simulink model "Deliverable2_SimulinkModel_Group37_Demo"  (R2023b)
settings: Solver=FixedStepAuto  StartTime=0.0  StopTime=10.0  RelTol=1e-3  EnableMultiTasking=on
undefined symbols (not defined in the file): A0, A1, D0, D1, D10, D11, D12, D13, D2, D3, D4, D5, D6, D7, D8, D9, PTA0, PTA1, PTA2, PTB2, PTB23, PTB3, PTB9, PTC16, PTC17, PTC2, PTC3, PTC4, PTD0, PTD1, PTD2, PTD3, send_params
libraries: frdmk64flib x20, etargetslib x2, simulink x2
settings Model: ExtModeTrigDuration=5  Creator=cakes  LastModifiedBy=cakes
settings OptimizationCC: EnhancedBackFolding=on  PassReuseOutputArgsAs=Individual arguments  ZeroExternalMemoryAtStartup=off  ZeroInternalMemoryAtStartup=off  MaxStackSize=64  OptimizeBlockOrder=speed  DifferentSizesBufferReuse=on  OptimizationCustomize=off  EfficientTunableParamExpr=on
settings DebuggingCC: ParameterTunabilityLossMsg=error
settings HardwareCC: ProdBitPerPointer=32  ProdBitPerSizeT=32  ProdBitPerPtrDiffT=32  ProdLargestAtomicInteger=Long  ProdLargestAtomicFloat=Double  ProdWordSize=32  ProdHWDeviceType=ARM Compatible->ARM Cortex
settings SFSimCC: MATLABDynamicMemAlloc=off
settings RTWCC: Description=Embedded Coder  SystemTargetFile=ert.tlc  HardwareBoard=NXP FRDM-K64F  TLCOptions="-aInlineSetEventsForThisBaseRateFcn=TLC_FALSE -aSuppressMultiTaskScheduler=TLC_FALSE  -aRateBasedStepFcn=0"  TemplateMakefile=ert_default_tmf  Toolchain=GNU Tools for ARM Embedded Processors
settings CodeAppCC: ForceParamTrailComments=on  IgnoreCustomStorageClasses=off  OperatorAnnotations=on  SimulinkDataObjDesc=on  SFDataObjDesc=on  InsertBlockDesc=on
settings ERTTargetCC: ExtModeTransport=4  ExtModeMexFile=sendToCommService

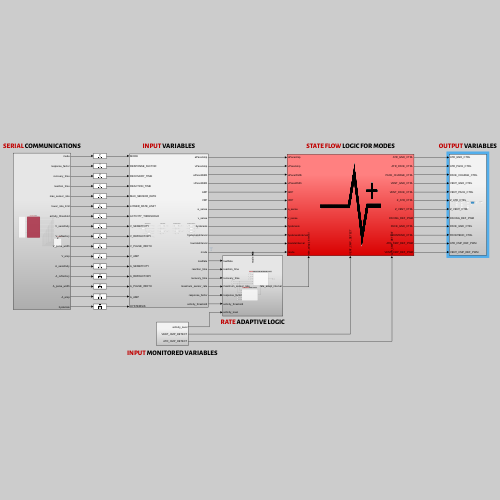
[thumbnail: Simulink's stored preview of the top-level diagram]
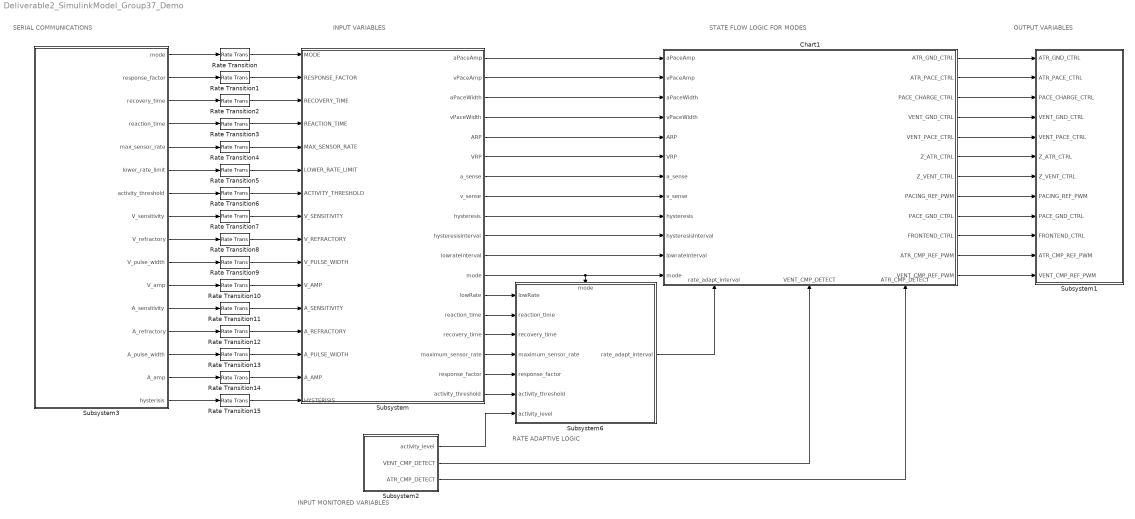
== system Deliverable2_SimulinkModel_Group37_Demo ==
  note: STATE FLOW LOGIC FOR MODES
  note: INPUT VARIABLES
  note: OUTPUT VARIABLES
  note: INPUT MONITORED VARIABLES
  note: SERIAL COMMUNICATIONS
  note: RATE ADAPTIVE LOGIC
  Chart1 : Stateflow chart  TreatAsAtomicUnit=on
      settings: PortSchema="{\"entries\":[{\"content\":{\"sides\":[{\"content\":{\"connectorIds\":[\"In3\",\"In4\",\"In5\",\"In6\",\"In7\",\"In8\",\"In10\",\"In11\",\"In14\",\"In13\",\"In9\",\"In12\"]},\"type\":\"ConnectorPlacement.EquallySpacedRectSide\",\"uuid\":\"0645b224-ea0f-4252-ab3f-59541b69d578\"},{\"content\":{\"connectorIds\":[\"Out1\",\"Out2\",\"Out3\",\"Out4\",\"Out5\",\"Out6\",\"Out7\",\"Out8\",\"Out9\",\"Out10\",\"Out12\",\"Out11\"],\"side\":\"RIGHT\"},\"type\":\"ConnectorPlacement.EquallySpacedRectSide\",\"uuid\":\"774839c9-1eb4-4ab6-be6e-099c2bb8a485\"},{\"content\":{\"side\":\"TOP\"},\"type\":\"ConnectorPlacement.EquallySpacedRectSide\",\"uuid\":\"6cb60565-1780-4b9d-884d-75d2ba8c5024\"},{\"content\":{\"connectorIds\":[\"In15\",\"In1\",\"In2\"],\"side\":\"BOTTOM\"},\"type\":\"ConnectorPlacement.EquallySpacedRectSide\",\"uuid\":\"cb44bc08-16a9-4dba-a42a-7ec56f3e5fd4\"}]},\"type\":\"ConnectorPlacement.EquallySpacedConnector\",\"uuid\":\"755e29d5-bc4e-404e-b866-950d5e4fdc89\"}],\"packageUris\":[\"http://schema.mathworks.com/mf0/Connector/R2020b\"],\"version\":\"1.0\"}"
  Rate Transition{,1..15} (16 alike) : RateTransition  OutPortSampleTime=0.001
  Subsystem : Subsystem
  Subsystem1 : Subsystem
  Subsystem2 : Subsystem
  Subsystem3 : Subsystem
  Subsystem6 : Subsystem
      settings: PortSchema="{\"entries\":[{\"content\":{\"sides\":[{\"content\":{\"connectorIds\":[\"In1\",\"In2\",\"In3\",\"In4\",\"In5\",\"In6\",\"In7\"]},\"type\":\"ConnectorPlacement.EquallySpacedRectSide\",\"uuid\":\"e8f7da03-bd10-42b0-9ffd-e59584e5bdf1\"},{\"content\":{\"connectorIds\":[\"Out1\"],\"side\":\"RIGHT\"},\"type\":\"ConnectorPlacement.EquallySpacedRectSide\",\"uuid\":\"86778467-52ef-4ae1-a721-8cc17c3ab00e\"},{\"content\":{\"connectorIds\":[\"In8\"],\"side\":\"TOP\"},\"type\":\"ConnectorPlacement.EquallySpacedRectSide\",\"uuid\":\"0329b3a8-8570-41f7-8001-3ae6aa58e01f\"}]},\"type\":\"ConnectorPlacement.EquallySpacedConnector\",\"uuid\":\"40165bd5-ab6e-4098-a980-e92209030f0d\"}],\"packageUris\":[\"http://schema.mathworks.com/mf0/Connector/R2020b\"],\"version\":\"1.0\"}"
  wires:
  Subsystem/1(aPaceAmp) -> Chart1/3(aPaceAmp)
  Subsystem/2(vPaceAmp) -> Chart1/4(vPaceAmp)
  Subsystem/3(aPaceWidth) -> Chart1/5(aPaceWidth)
  Subsystem/4(vPaceWidth) -> Chart1/6(vPaceWidth)
  Subsystem/5(ARP) -> Chart1/7(ARP)
  Subsystem/6(VRP) -> Chart1/8(VRP)
  Subsystem/11(lowrateInterval) -> Chart1/9(lowrateInterval)
  Subsystem/12(mode) -> Subsystem6/8(mode), Chart1/12(mode)
  Chart1/1(ATR_GND_CTRL) -> Subsystem1/1(ATR_GND_CTRL)
  Chart1/2(ATR_PACE_CTRL) -> Subsystem1/2(ATR_PACE_CTRL)
  Chart1/3(PACE_CHARGE_CTRL) -> Subsystem1/3(PACE_CHARGE_CTRL)
  Chart1/4(VENT_GND_CTRL) -> Subsystem1/4(VENT_GND_CTRL)
  Chart1/5(VENT_PACE_CTRL) -> Subsystem1/5(VENT_PACE_CTRL)
  Chart1/6(Z_ATR_CTRL) -> Subsystem1/6(Z_ATR_CTRL)
  Subsystem2/2(VENT_CMP_DETECT) -> Chart1/1(VENT_CMP_DETECT)
  Chart1/9(PACE_GND_CTRL) -> Subsystem1/9(PACE_GND_CTRL)
  Subsystem/7(a_sense) -> Chart1/10(a_sense)
  Subsystem/8(v_sense) -> Chart1/11(v_sense)
  Chart1/10(FRONTEND_CTRL) -> Subsystem1/10(FRONTEND_CTRL)
  Chart1/11(VENT_CMP_REF_PWM) -> Subsystem1/12(VENT_CMP_REF_PWM)
  Chart1/7(Z_VENT_CTRL) -> Subsystem1/7(Z_VENT_CTRL)
  Chart1/8(PACING_REF_PWM) -> Subsystem1/8(PACING_REF_PWM)
  Chart1/12(ATR_CMP_REF_PWM) -> Subsystem1/11(ATR_CMP_REF_PWM)
  Subsystem2/3(ATR_CMP_DETECT) -> Chart1/2(ATR_CMP_DETECT)
  Subsystem/9(hysteresis) -> Chart1/14(hysteresis)
  Subsystem/10(hysteresisInterval) -> Chart1/13(hysteresisInterval)
  Subsystem/17(response_factor) -> Subsystem6/5(response_factor)
  Subsystem/16(maximum_sensor_rate) -> Subsystem6/4(maximum_sensor_rate)
  Subsystem/13(lowRate) -> Subsystem6/1(lowRate)
  Subsystem/14(reaction_time) -> Subsystem6/2(reaction_time)
  Subsystem/15(recovery_time) -> Subsystem6/3(recovery_time)
  Subsystem/18(activity_threshold) -> Subsystem6/6(activity_threshold)
  Subsystem6/1(rate_adapt_interval) -> Chart1/15(rate_adapt_interval)
  Subsystem2/1(activity_level) -> Subsystem6/7(activity_level)
  Subsystem3/1(mode) -> Rate Transition/1
  Subsystem3/2(response_factor) -> Rate Transition1/1
  Subsystem3/3(recovery_time) -> Rate Transition2/1
  Subsystem3/4(reaction_time) -> Rate Transition3/1
  Subsystem3/5(max_sensor_rate) -> Rate Transition4/1
  Subsystem3/7(activity_threshold) -> Rate Transition6/1
  Subsystem3/8(V_sensitivity) -> Rate Transition7/1
  Subsystem3/9(V_refractory) -> Rate Transition8/1
  Subsystem3/10(V_pulse_width) -> Rate Transition9/1
  Subsystem3/14(A_pulse_width) -> Rate Transition13/1
  Subsystem3/13(A_refractory) -> Rate Transition12/1
  Subsystem3/12(A_sensitivity) -> Rate Transition11/1
  Subsystem3/11(V_amp) -> Rate Transition10/1
  Subsystem3/15(A_amp) -> Rate Transition14/1
  Subsystem3/16(hysterisis) -> Rate Transition15/1
  Subsystem3/6(lower_rate_limit) -> Rate Transition5/1
  Rate Transition/1 -> Subsystem/1(MODE)
  Rate Transition1/1 -> Subsystem/2(RESPONSE_FACTOR)
  Rate Transition3/1 -> Subsystem/4(REACTION_TIME)
  Rate Transition2/1 -> Subsystem/3(RECOVERY_TIME)
  Rate Transition4/1 -> Subsystem/5(MAX_SENSOR_RATE)
  Rate Transition5/1 -> Subsystem/6(LOWER_RATE_LIMIT)
  Rate Transition7/1 -> Subsystem/8(V_SENSITIVITY)
  Rate Transition6/1 -> Subsystem/7(ACTIVITY_THRESHOLD)
  Rate Transition9/1 -> Subsystem/10(V_PULSE_WIDTH)
  Rate Transition8/1 -> Subsystem/9(V_REFRACTORY)
  Rate Transition11/1 -> Subsystem/12(A_SENSITIVITY)
  Rate Transition10/1 -> Subsystem/11(V_AMP)
  Rate Transition13/1 -> Subsystem/14(A_PULSE_WIDTH)
  Rate Transition14/1 -> Subsystem/15(A_AMP)
  Rate Transition12/1 -> Subsystem/13(A_REFRACTORY)
  Rate Transition15/1 -> Subsystem/16(HYSTERISIS)

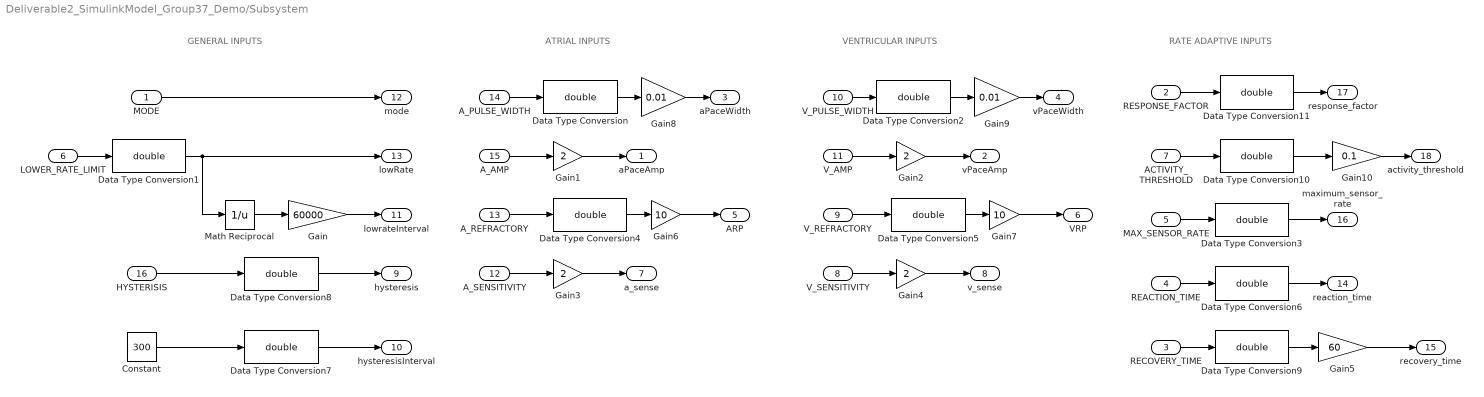
== system Deliverable2_SimulinkModel_Group37_Demo/Subsystem ==
  note: GENERAL INPUTS
  note: ATRIAL INPUTS
  note: VENTRICULAR INPUTS
  note: RATE ADAPTIVE INPUTS
  MODE : Inport
  RESPONSE_FACTOR : Inport  Port=2
  RECOVERY_TIME : Inport  Port=3
  REACTION_TIME : Inport  Port=4
  MAX_SENSOR_RATE : Inport  Port=5
  LOWER_RATE_LIMIT : Inport  Port=6
  ACTIVITY_THRESHOLD : Inport  Port=7
  V_SENSITIVITY : Inport  Port=8
  V_REFRACTORY : Inport  Port=9
  V_PULSE_WIDTH : Inport  Port=10
  V_AMP : Inport  Port=11
  A_SENSITIVITY : Inport  Port=12
  A_REFRACTORY : Inport  Port=13
  A_PULSE_WIDTH : Inport  Port=14
  A_AMP : Inport  Port=15
  HYSTERISIS : Inport  Port=16
  Constant : Constant  Value=300
  Data Type Conversion{,1..11} (12 alike) : DataTypeConversion  OutDataTypeStr=double  SaturateOnIntegerOverflow=off  RndMeth=Floor
  Gain : Gain  Gain=60000
  Gain1 : Gain  Gain=2  OutDataTypeStr=double
  Gain10 : Gain  Gain=0.1  OutDataTypeStr=double
  Gain2 : Gain  Gain=2  OutDataTypeStr=double
  Gain3 : Gain  Gain=2
  Gain4 : Gain  Gain=2
  Gain5 : Gain  Gain=60  OutDataTypeStr=double
  Gain6 : Gain  Gain=10  OutDataTypeStr=double
  Gain7 : Gain  Gain=10  OutDataTypeStr=double
  Gain8 : Gain  Gain=0.01  OutDataTypeStr=double
  Gain9 : Gain  Gain=0.01  OutDataTypeStr=double
  Math Reciprocal : Math  Operator=reciprocal  SignedPower=on
  aPaceAmp : Outport
  vPaceAmp : Outport  Port=2
  aPaceWidth : Outport  Port=3
  vPaceWidth : Outport  Port=4
  ARP : Outport  Port=5
  VRP : Outport  Port=6
  a_sense : Outport  Port=7
  v_sense : Outport  Port=8
  hysteresis : Outport  Port=9
  hysteresisInterval : Outport  Port=10
  lowrateInterval : Outport  Port=11
  mode : Outport  Port=12
  lowRate : Outport  Port=13
  reaction_time : Outport  Port=14
  recovery_time : Outport  Port=15
  maximum_sensor_rate : Outport  Port=16
  response_factor : Outport  Port=17
  activity_threshold : Outport  Port=18
  wires:
  A_PULSE_WIDTH/1 -> Data Type Conversion/1
  V_PULSE_WIDTH/1 -> Data Type Conversion2/1
  MODE/1 -> mode/1
  HYSTERISIS/1 -> Data Type Conversion8/1
  Constant/1 -> Data Type Conversion7/1
  Math Reciprocal/1 -> Gain/1
  Gain1/1 -> aPaceAmp/1
  Gain2/1 -> vPaceAmp/1
  A_SENSITIVITY/1 -> Gain3/1
  V_SENSITIVITY/1 -> Gain4/1
  Gain4/1 -> v_sense/1
  Gain3/1 -> a_sense/1
  RESPONSE_FACTOR/1 -> Data Type Conversion11/1
  RECOVERY_TIME/1 -> Data Type Conversion9/1
  Gain5/1 -> recovery_time/1
  MAX_SENSOR_RATE/1 -> Data Type Conversion3/1
  Data Type Conversion3/1 -> maximum_sensor_rate/1
  Data Type Conversion6/1 -> reaction_time/1
  A_REFRACTORY/1 -> Data Type Conversion4/1
  Gain6/1 -> ARP/1
  V_REFRACTORY/1 -> Data Type Conversion5/1
  Gain7/1 -> VRP/1
  Gain/1 -> lowrateInterval/1
  Data Type Conversion1/1 -> Math Reciprocal/1, lowRate/1
  LOWER_RATE_LIMIT/1 -> Data Type Conversion1/1
  A_AMP/1 -> Gain1/1
  V_AMP/1 -> Gain2/1
  Data Type Conversion4/1 -> Gain6/1
  Data Type Conversion5/1 -> Gain7/1
  REACTION_TIME/1 -> Data Type Conversion6/1
  Data Type Conversion7/1 -> hysteresisInterval/1
  Data Type Conversion8/1 -> hysteresis/1
  Data Type Conversion/1 -> Gain8/1
  Gain8/1 -> aPaceWidth/1
  Gain9/1 -> vPaceWidth/1
  Data Type Conversion2/1 -> Gain9/1
  Data Type Conversion9/1 -> Gain5/1
  Data Type Conversion11/1 -> response_factor/1
  ACTIVITY_THRESHOLD/1 -> Data Type Conversion10/1
  Data Type Conversion10/1 -> Gain10/1
  Gain10/1 -> activity_threshold/1

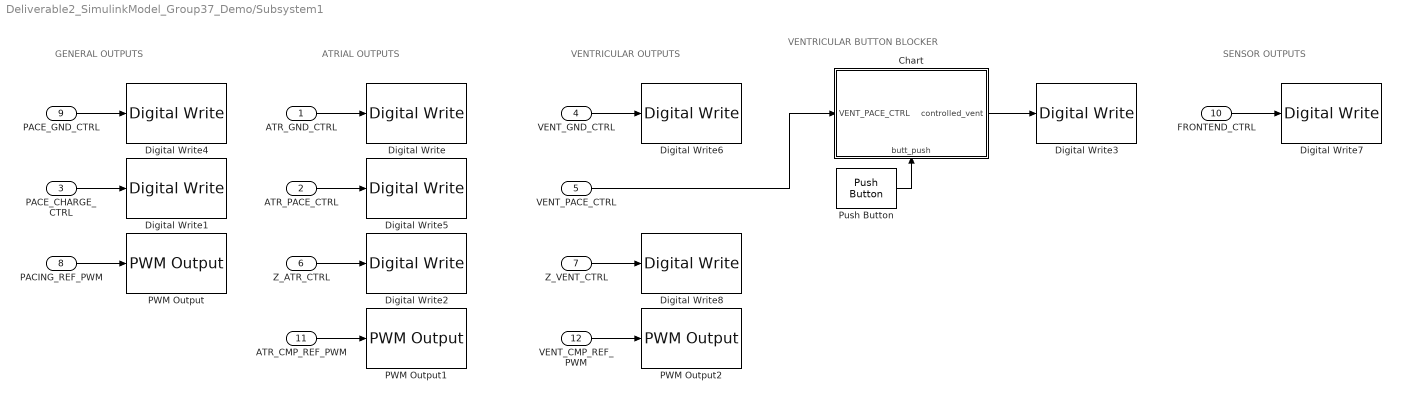
== system Deliverable2_SimulinkModel_Group37_Demo/Subsystem1 ==
  note: ATRIAL OUTPUTS
  note: GENERAL OUTPUTS
  note: VENTRICULAR OUTPUTS
  note: SENSOR OUTPUTS
  note: VENTRICULAR BUTTON BLOCKER
  ATR_GND_CTRL : Inport
  ATR_PACE_CTRL : Inport  Port=2
  PACE_CHARGE_CTRL : Inport  Port=3
  VENT_GND_CTRL : Inport  Port=4
  VENT_PACE_CTRL : Inport  Port=5
  Z_ATR_CTRL : Inport  Port=6
  Z_VENT_CTRL : Inport  Port=7
  PACING_REF_PWM : Inport  Port=8
  PACE_GND_CTRL : Inport  Port=9
  FRONTEND_CTRL : Inport  Port=10
  ATR_CMP_REF_PWM : Inport  Port=11
  VENT_CMP_REF_PWM : Inport  Port=12
  Chart : Stateflow chart  TreatAsAtomicUnit=on
      settings: PortSchema="{\"entries\":[{\"content\":{\"sides\":[{\"content\":{\"connectorIds\":[\"In2\"]},\"type\":\"ConnectorPlacement.EquallySpacedRectSide\",\"uuid\":\"797f1e7f-6824-45b0-bf45-566c15de680c\"},{\"content\":{\"connectorIds\":[\"Out1\"],\"side\":\"RIGHT\"},\"type\":\"ConnectorPlacement.EquallySpacedRectSide\",\"uuid\":\"8412beb8-8a5e-4913-a0e4-357c6aa96866\"},{\"content\":{\"side\":\"TOP\"},\"type\":\"ConnectorPlacement.EquallySpacedRectSide\",\"uuid\":\"c81022a9-b08e-44c9-8a82-e62bdb07cf60\"},{\"content\":{\"connectorIds\":[\"In1\"],\"side\":\"BOTTOM\"},\"type\":\"ConnectorPlacement.EquallySpacedRectSide\",\"uuid\":\"3d859f7f-1411-4a74-b08f-b013bf866652\"}]},\"type\":\"ConnectorPlacement.EquallySpacedConnector\",\"uuid\":\"ada65d55-343c-44f5-81cf-1c10e0b2b42c\"}],\"packageUris\":[\"http://schema.mathworks.com/mf0/Connector/R2020b\"],\"version\":\"1.0\"}"
  Digital Write : frdmk64flib/Digital Write  Whichpin=PTD2 (D11)
  Digital Write1 : frdmk64flib/Digital Write  Whichpin=PTB9 (D2)
  Digital Write2 : frdmk64flib/Digital Write  Whichpin=PTB23 (D4)
  Digital Write3 : frdmk64flib/Digital Write  Whichpin=PTC4 (D9)
  Digital Write4 : frdmk64flib/Digital Write  Whichpin=PTD0 (D10)
  Digital Write5 : frdmk64flib/Digital Write  Whichpin=PTA0 (D8)
  Digital Write6 : frdmk64flib/Digital Write  Whichpin=PTD3 (D12)
  Digital Write7 : frdmk64flib/Digital Write  Whichpin=PTD1 (D13)
  Digital Write8 : frdmk64flib/Digital Write  Whichpin=PTC3 (D7)
  PWM Output : frdmk64flib/PWM Output  Whichpin=PTA2 (D5)  InitialFrequency=2000  InitialDutyCycle=0
  PWM Output1 : frdmk64flib/PWM Output  Whichpin=PTC2 (D6)  InitialFrequency=2000  InitialDutyCycle=0
  PWM Output2 : frdmk64flib/PWM Output  Whichpin=PTA1 (D3)  InitialFrequency=2000  InitialDutyCycle=0
  Push Button : frdmk64flib/Push Button  Whichswitch=SW2  SampleTime1=-1
  wires:
  PACING_REF_PWM/1 -> PWM Output/1
  Z_ATR_CTRL/1 -> Digital Write2/1
  PACE_CHARGE_CTRL/1 -> Digital Write1/1
  ATR_PACE_CTRL/1 -> Digital Write5/1
  ATR_GND_CTRL/1 -> Digital Write/1
  VENT_GND_CTRL/1 -> Digital Write6/1
  FRONTEND_CTRL/1 -> Digital Write7/1
  Z_VENT_CTRL/1 -> Digital Write8/1
  PACE_GND_CTRL/1 -> Digital Write4/1
  ATR_CMP_REF_PWM/1 -> PWM Output1/1
  VENT_CMP_REF_PWM/1 -> PWM Output2/1
  VENT_PACE_CTRL/1 -> Chart/2(VENT_PACE_CTRL)
  Push Button/1 -> Chart/1(butt_push)
  Chart/1(controlled_vent) -> Digital Write3/1

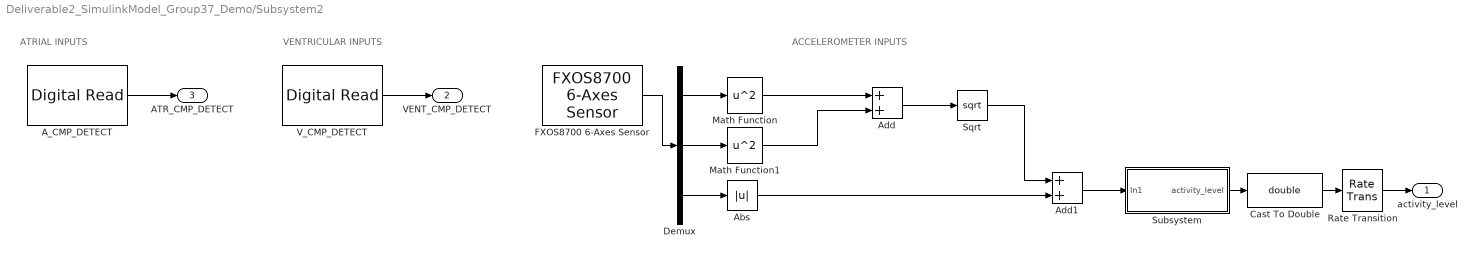
== system Deliverable2_SimulinkModel_Group37_Demo/Subsystem2 ==
  note: ATRIAL INPUTS
  note: VENTRICULAR INPUTS
  note: ACCELEROMETER INPUTS
  A_CMP_DETECT : frdmk64flib/Digital Read  Whichpin=PTC16 (D0)  SampleTime=0.001
  Abs : Abs  SaturateOnIntegerOverflow=off
  Add : Sum
  Add1 : Sum
  Cast To Double : DataTypeConversion  OutDataTypeStr=double  SaturateOnIntegerOverflow=off  RndMeth=Floor
  Demux : Demux  Outputs=3
  FXOS8700 6-Axes Sensor : frdmk64flib/FXOS8700 6-Axes Sensor  Activesensor=Accelerometer only  ODR=50Hz  HybridODR=400Hz  Accelfullrange=-4g to +4g  SampleTime=0.01
  Math Function : Math  Operator=square
  Math Function1 : Math  Operator=square
  Rate Transition : RateTransition  OutPortSampleTime=0.001
  Sqrt : Sqrt
  Subsystem : Subsystem
  V_CMP_DETECT : frdmk64flib/Digital Read  Whichpin=PTC17 (D1)  SampleTime=0.001
  activity_level : Outport
  VENT_CMP_DETECT : Outport  Port=2
  ATR_CMP_DETECT : Outport  Port=3
  wires:
  V_CMP_DETECT/1 -> VENT_CMP_DETECT/1
  A_CMP_DETECT/1 -> ATR_CMP_DETECT/1
  FXOS8700 6-Axes Sensor/1 -> Demux/1
  Add/1 -> Sqrt/1
  Add1/1 -> Subsystem/1(In1)
  Demux/3 -> Abs/1
  Demux/1 -> Math Function/1
  Subsystem/1(activity_level) -> Cast To Double/1
  Sqrt/1 -> Add1/1
  Abs/1 -> Add1/2
  Math Function1/1 -> Add/2
  Math Function/1 -> Add/1
  Demux/2 -> Math Function1/1
  Rate Transition/1 -> activity_level/1
  Cast To Double/1 -> Rate Transition/1

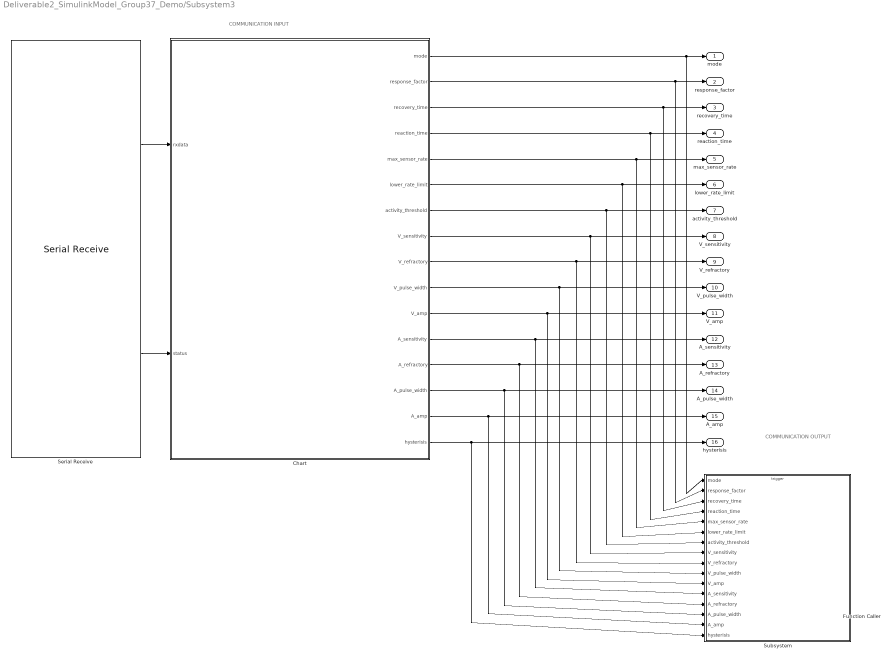
== system Deliverable2_SimulinkModel_Group37_Demo/Subsystem3 ==
  note: COMMUNICATION OUTPUT
  note: COMMUNICATION INPUT
  Chart : Stateflow chart  TreatAsAtomicUnit=on
  Function Caller : FunctionCaller  FunctionPrototype=send_params()  InputArgumentSpecifications=<Enter example>  OutputArgumentSpecifications=<Enter example>  SampleTime=0.01
  Serial Receive : frdmk64flib/Serial Receive  SCIModule=0  Baudrate=uint32(9600)  Parity=None  StopBits=1  HardwareFlowControl=None  ByteOrder=LittleEndian  DataType=uint8  DataLength=18  BlockingMode=off  OutputStatus=on  SampleTime=0.01
  Subsystem : Subsystem
  mode : Outport
  response_factor : Outport  Port=2
  recovery_time : Outport  Port=3
  reaction_time : Outport  Port=4
  max_sensor_rate : Outport  Port=5
  lower_rate_limit : Outport  Port=6
  activity_threshold : Outport  Port=7
  V_sensitivity : Outport  Port=8
  V_refractory : Outport  Port=9
  V_pulse_width : Outport  Port=10
  V_amp : Outport  Port=11
  A_sensitivity : Outport  Port=12
  A_refractory : Outport  Port=13
  A_pulse_width : Outport  Port=14
  A_amp : Outport  Port=15
  hysterisis : Outport  Port=16
  wires:
  Serial Receive/1 -> Chart/1(rxdata)
  Serial Receive/2 -> Chart/2(status)
  Chart/1(mode) -> Subsystem/1(mode), mode/1
  Chart/3(recovery_time) -> Subsystem/3(recovery_time), recovery_time/1
  Chart/4(reaction_time) -> Subsystem/4(reaction_time), reaction_time/1
  Chart/5(max_sensor_rate) -> Subsystem/5(max_sensor_rate), max_sensor_rate/1
  Chart/6(lower_rate_limit) -> Subsystem/6(lower_rate_limit), lower_rate_limit/1
  Chart/7(activity_threshold) -> Subsystem/7(activity_threshold), activity_threshold/1
  Chart/8(V_sensitivity) -> Subsystem/8(V_sensitivity), V_sensitivity/1
  Chart/9(V_refractory) -> Subsystem/9(V_refractory), V_refractory/1
  Chart/10(V_pulse_width) -> Subsystem/10(V_pulse_width), V_pulse_width/1
  Chart/11(V_amp) -> Subsystem/11(V_amp), V_amp/1
  Chart/12(A_sensitivity) -> A_sensitivity/1, Subsystem/12(A_sensitivity)
  Chart/13(A_refractory) -> A_refractory/1, Subsystem/13(A_refractory)
  Chart/14(A_pulse_width) -> A_pulse_width/1, Subsystem/14(A_pulse_width)
  Chart/15(A_amp) -> A_amp/1, Subsystem/15(A_amp)
  Chart/16(hysterisis) -> hysterisis/1, Subsystem/16(hysterisis)
  Chart/2(response_factor) -> Subsystem/2(response_factor), response_factor/1

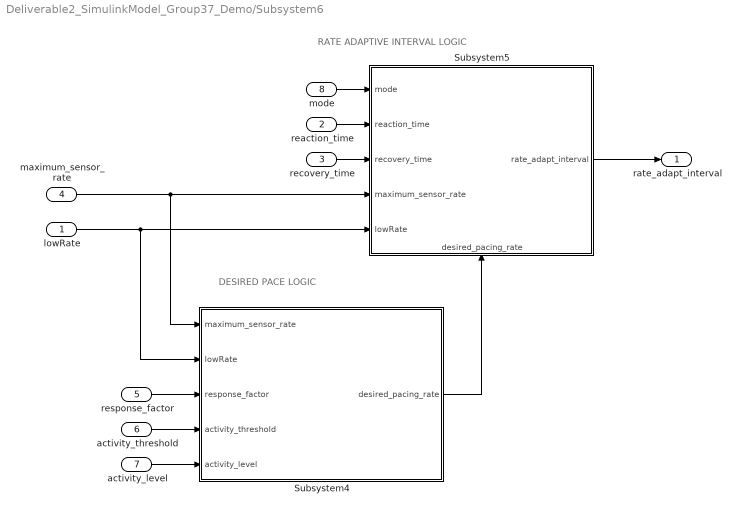
== system Deliverable2_SimulinkModel_Group37_Demo/Subsystem6 ==
  note: DESIRED PACE LOGIC
  note: RATE ADAPTIVE INTERVAL LOGIC
  lowRate : Inport
  reaction_time : Inport  Port=2
  recovery_time : Inport  Port=3
  maximum_sensor_rate : Inport  Port=4
  response_factor : Inport  Port=5
  activity_threshold : Inport  Port=6
  activity_level : Inport  Port=7
  mode : Inport  Port=8
  Subsystem4 : Subsystem
  Subsystem5 : Subsystem
      settings: PortSchema="{\"entries\":[{\"content\":{\"sides\":[{\"content\":{\"connectorIds\":[\"In1\",\"In2\",\"In3\",\"In4\",\"In5\"]},\"type\":\"ConnectorPlacement.EquallySpacedRectSide\",\"uuid\":\"79bc3fb3-9fea-4441-ae48-8f2cb8dc5d6d\"},{\"content\":{\"connectorIds\":[\"Out1\"],\"side\":\"RIGHT\"},\"type\":\"ConnectorPlacement.EquallySpacedRectSide\",\"uuid\":\"8e25f63d-7a7f-4a30-9d51-ff4e93a9aa99\"},{\"content\":{\"side\":\"TOP\"},\"type\":\"ConnectorPlacement.EquallySpacedRectSide\",\"uuid\":\"e07be596-e475-4181-9b08-2e1f9ea03076\"},{\"content\":{\"connectorIds\":[\"In6\"],\"side\":\"BOTTOM\"},\"type\":\"ConnectorPlacement.EquallySpacedRectSide\",\"uuid\":\"37a509d1-15c0-445b-9b56-eefd17d0fdfa\"}]},\"type\":\"ConnectorPlacement.EquallySpacedConnector\",\"uuid\":\"3beff34e-2a6c-47b3-9523-1069d662617f\"}],\"packageUris\":[\"http://schema.mathworks.com/mf0/Connector/R2020b\"],\"version\":\"1.0\"}"
  rate_adapt_interval : Outport
  wires:
  Subsystem5/1(rate_adapt_interval) -> rate_adapt_interval/1
  reaction_time/1 -> Subsystem5/2(reaction_time)
  recovery_time/1 -> Subsystem5/3(recovery_time)
  maximum_sensor_rate/1 -> Subsystem4/1(maximum_sensor_rate), Subsystem5/4(maximum_sensor_rate)
  lowRate/1 -> Subsystem4/2(lowRate), Subsystem5/5(lowRate)
  activity_threshold/1 -> Subsystem4/4(activity_threshold)
  response_factor/1 -> Subsystem4/3(response_factor)
  activity_level/1 -> Subsystem4/5(activity_level)
  Subsystem4/1(desired_pacing_rate) -> Subsystem5/6(desired_pacing_rate)
  mode/1 -> Subsystem5/1(mode)

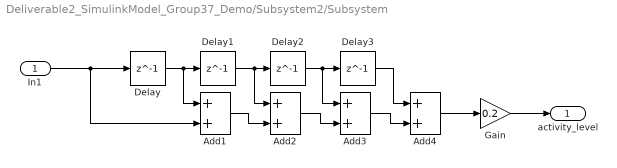
== system Deliverable2_SimulinkModel_Group37_Demo/Subsystem2/Subsystem ==
  In1 : Inport
  Add{1..4} (4 alike) : Sum
  Delay{,1..3} (4 alike) : Delay  DelayLength=1
  Gain : Gain  Gain=0.2
  activity_level : Outport
  wires:
  Delay/1 -> Add1/1, Delay1/1
  Delay1/1 -> Add2/1, Delay2/1
  Delay2/1 -> Add3/1, Delay3/1
  In1/1 -> Delay/1, Add1/2
  Add1/1 -> Add2/2
  Add4/1 -> Gain/1
  Add2/1 -> Add3/2
  Add3/1 -> Add4/2
  Delay3/1 -> Add4/1
  Gain/1 -> activity_level/1

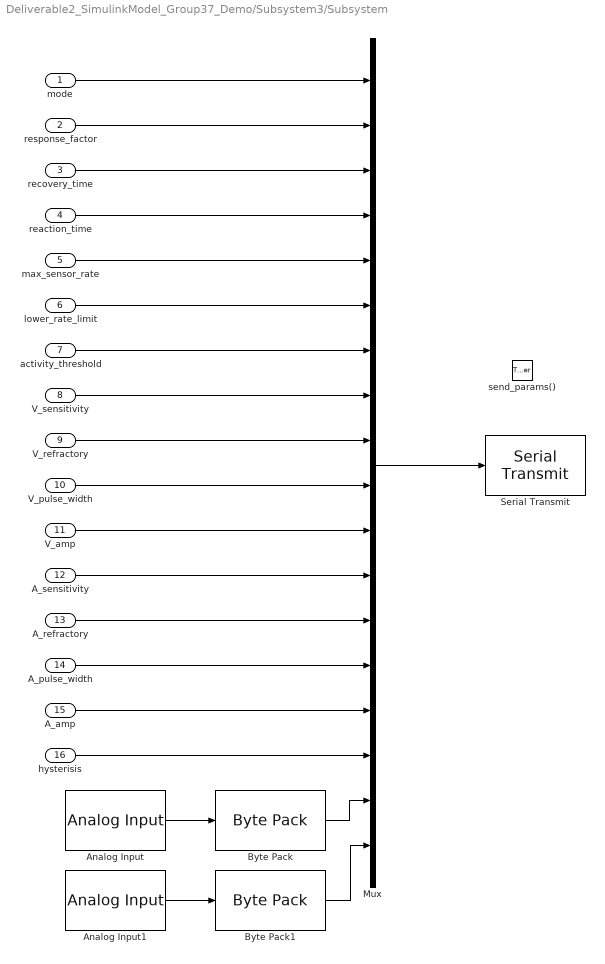
== system Deliverable2_SimulinkModel_Group37_Demo/Subsystem3/Subsystem ==
  mode : Inport
  response_factor : Inport  Port=2
  recovery_time : Inport  Port=3
  reaction_time : Inport  Port=4
  max_sensor_rate : Inport  Port=5
  lower_rate_limit : Inport  Port=6
  activity_threshold : Inport  Port=7
  V_sensitivity : Inport  Port=8
  V_refractory : Inport  Port=9
  V_pulse_width : Inport  Port=10
  V_amp : Inport  Port=11
  A_sensitivity : Inport  Port=12
  A_refractory : Inport  Port=13
  A_pulse_width : Inport  Port=14
  A_amp : Inport  Port=15
  hysterisis : Inport  Port=16
  send_params() : TriggerPort  TriggerType=function-call  IsSimulinkFunction=on  FunctionName=send_params  VariantControl=(inherit)  PortDimensions=1
  Analog Input : frdmk64flib/Analog Input  Whichpin=PTB2 (A0)  SampleTime=-1
  Analog Input1 : frdmk64flib/Analog Input  Whichpin=PTB3 (A1)  SampleTime=-1
  Byte Pack : etargetslib/Byte Pack  datatypes={'double'}  byteAlign=1
  Byte Pack1 : etargetslib/Byte Pack  datatypes={'double'}  byteAlign=1
  Mux : Mux  Inputs=18
  Serial Transmit : frdmk64flib/Serial Transmit  SCIModule=0  Baudrate=uint32(9600)  Parity=None  StopBits=1  HardwareFlowControl=None  ByteOrder=LittleEndian  BlockingMode=on  OutputStatus=off
  wires:
  Mux/1 -> Serial Transmit/1
  mode/1 -> Mux/1
  response_factor/1 -> Mux/2
  recovery_time/1 -> Mux/3
  reaction_time/1 -> Mux/4
  max_sensor_rate/1 -> Mux/5
  lower_rate_limit/1 -> Mux/6
  activity_threshold/1 -> Mux/7
  V_sensitivity/1 -> Mux/8
  V_refractory/1 -> Mux/9
  V_pulse_width/1 -> Mux/10
  V_amp/1 -> Mux/11
  A_sensitivity/1 -> Mux/12
  A_refractory/1 -> Mux/13
  A_pulse_width/1 -> Mux/14
  A_amp/1 -> Mux/15
  hysterisis/1 -> Mux/16
  Analog Input/1 -> Byte Pack/1
  Analog Input1/1 -> Byte Pack1/1
  Byte Pack/1 -> Mux/17
  Byte Pack1/1 -> Mux/18

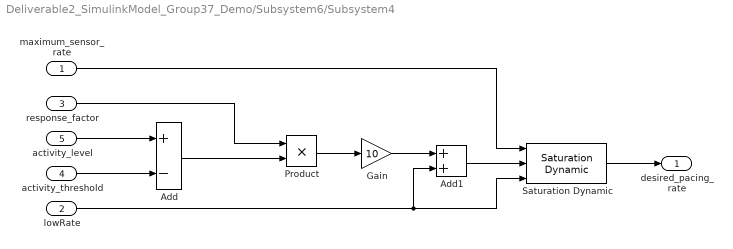
== system Deliverable2_SimulinkModel_Group37_Demo/Subsystem6/Subsystem4 ==
  maximum_sensor_rate : Inport
  lowRate : Inport  Port=2
  response_factor : Inport  Port=3
  activity_threshold : Inport  Port=4
  activity_level : Inport  Port=5
  Add : Sum  Inputs=+-
  Add1 : Sum
  Gain : Gain  Gain=10
  Product : Product
  Saturation Dynamic : simulink/Discontinuities/Saturation Dynamic  OutMin=[]  OutMax=[]  OutDataTypeStr=double  OutDataType=fixdt(1, 16)  OutScaling=2^-10  RndMeth=Nearest  DoSatur=off
  desired_pacing_rate : Outport
  wires:
  activity_level/1 -> Add/1
  activity_threshold/1 -> Add/2
  Add/1 -> Product/2
  response_factor/1 -> Product/1
  Gain/1 -> Add1/1
  Product/1 -> Gain/1
  lowRate/1 -> Saturation Dynamic/3, Add1/2
  Add1/1 -> Saturation Dynamic/2
  maximum_sensor_rate/1 -> Saturation Dynamic/1
  Saturation Dynamic/1 -> desired_pacing_rate/1

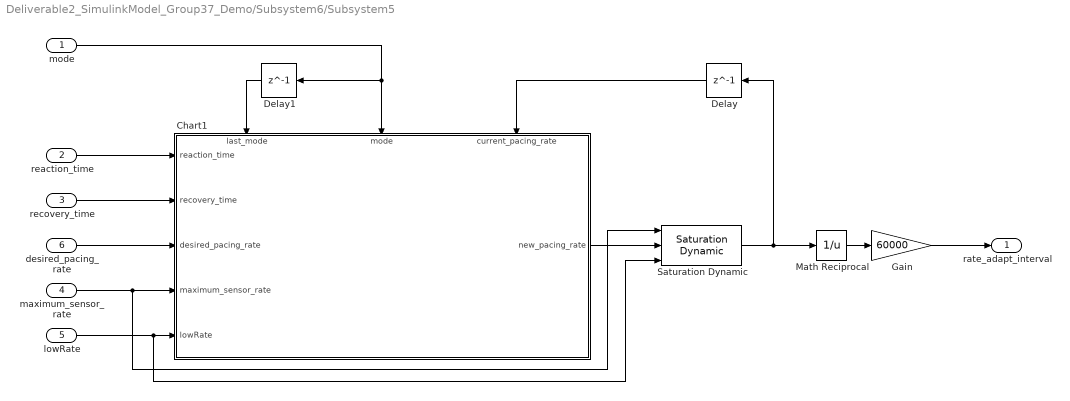
== system Deliverable2_SimulinkModel_Group37_Demo/Subsystem6/Subsystem5 ==
  mode : Inport
  reaction_time : Inport  Port=2
  recovery_time : Inport  Port=3
  maximum_sensor_rate : Inport  Port=4
  lowRate : Inport  Port=5
  desired_pacing_rate : Inport  Port=6
  Chart1 : Stateflow chart  TreatAsAtomicUnit=on
      settings: PortSchema="{\"entries\":[{\"content\":{\"sides\":[{\"content\":{\"connectorIds\":[\"In4\",\"In5\",\"In6\",\"In8\",\"In7\"]},\"type\":\"ConnectorPlacement.EquallySpacedRectSide\",\"uuid\":\"06a0217b-4288-43b0-8932-705b4d4ece1e\"},{\"content\":{\"connectorIds\":[\"Out1\"],\"side\":\"RIGHT\"},\"type\":\"ConnectorPlacement.EquallySpacedRectSide\",\"uuid\":\"c8eefe2e-d095-40c8-acb0-aebaf19a9365\"},{\"content\":{\"connectorIds\":[\"In2\",\"In1\",\"In3\"],\"side\":\"TOP\"},\"type\":\"ConnectorPlacement.EquallySpacedRectSide\",\"uuid\":\"128ffed5-e0e5-4f4f-9131-f15ad41e2462\"},{\"content\":{\"side\":\"BOTTOM\"},\"type\":\"ConnectorPlacement.EquallySpacedRectSide\",\"uuid\":\"a7475944-bf84-45a0-8219-ddf2a50d7d23\"}]},\"type\":\"ConnectorPlacement.EquallySpacedConnector\",\"uuid\":\"00626f3d-df19-4fc7-9d9d-9a6ae210b908\"}],\"packageUris\":[\"http://schema.mathworks.com/mf0/Connector/R2020b\"],\"version\":\"1.0\"}"
  Delay : Delay  DelayLength=1  InitialCondition=60
  Delay1 : Delay  DelayLength=1  InitialCondition=60
  Gain : Gain  Gain=60000  OutDataTypeStr=double
  Math Reciprocal : Math  Operator=reciprocal  SignedPower=on
  Saturation Dynamic : simulink/Discontinuities/Saturation Dynamic  OutMin=[]  OutMax=[]  OutDataTypeStr=double  OutDataType=fixdt(1, 16)  OutScaling=2^-10  RndMeth=Nearest  DoSatur=off
  rate_adapt_interval : Outport
  wires:
  Math Reciprocal/1 -> Gain/1
  reaction_time/1 -> Chart1/4(reaction_time)
  Delay/1 -> Chart1/3(current_pacing_rate)
  maximum_sensor_rate/1 -> Chart1/8(maximum_sensor_rate), Saturation Dynamic/1
  recovery_time/1 -> Chart1/5(recovery_time)
  lowRate/1 -> Chart1/7(lowRate), Saturation Dynamic/3
  desired_pacing_rate/1 -> Chart1/6(desired_pacing_rate)
  Gain/1 -> rate_adapt_interval/1
  Saturation Dynamic/1 -> Math Reciprocal/1, Delay/1
  Chart1/1(new_pacing_rate) -> Saturation Dynamic/2
  Delay1/1 -> Chart1/2(last_mode)
  mode/1 -> Delay1/1, Chart1/1(mode)

== stateflow chart Deliverable2_SimulinkModel_Group37_Demo/Chart1 ==
  settings: sampleTime=0.001
  state INIT
    entry:
    %inital state, reset variables when mode change
    PACE_CHARGE_CTRL = 0;
    ATR_PACE_CTRL = 0;
    ATR_GND_CTRL = 0;
    VENT_PACE_CTRL=0;
    VENT_GND_CTRL=0;
    Z_ATR_CTRL = 0;
    Z_VENT_CTRL=0;
    PACE_GND_CTRL=0;
    PACING_REF_PWM=0;
    PACE_CHARGE_CTRL=0;
    FRONTEND_CTRL =1;
    VENT_CMP_REF_PWM = v_sense;
    ATR_CMP_REF_PWM = a_sense;
    note: MODE
        | NUMBER
        |
        | AOO
        | 0
        |
        | VOO
        | 1
        |
        | AAI
        | 2
        |
        | VVI
        | 3
        |
        | AOOR
        | 4
        |
        | VOOR
        | 5
        |
        | AAIR
        | 6
        |
        | VVIR
        | 7
        |
        | DDR
        | 8
  state AOO
    state AOO_Charging
      %charging capacitor
      entry:
      PACING_REF_PWM = aPaceAmp;
      PACE_GND_CTRL = 1;
      Z_ATR_CTRL = 0;
      ATR_PACE_CTRL = 0;
      PACE_CHARGE_CTRL = 1;
      ATR_GND_CTRL = 1;
    state AOO_Pacing
      %discharging
      entry:
      Z_ATR_CTRL = 1;
      PACE_CHARGE_CTRL = 0;
      ATR_GND_CTRL = 0;
      ATR_PACE_CTRL = 1;
    (default) -> AOO_Charging
    AOO_Charging -> AOO_Pacing : after(lowrateInterval - aPaceWidth, msec)
    AOO_Pacing -> AOO_Charging : after(aPaceWidth, msec)
  state VOO
    state VOO_Charging
      %charging capacitor
      entry:
      PACING_REF_PWM = vPaceAmp;
      PACE_GND_CTRL = 1;
      Z_VENT_CTRL = 0;
      VENT_PACE_CTRL = 0;
      PACE_CHARGE_CTRL = 1;
      VENT_GND_CTRL = 1;
    state VOO_Pacing
      %discharging capacitor
      entry:
      Z_VENT_CTRL = 1;
      PACE_CHARGE_CTRL = 0;
      VENT_GND_CTRL = 0;
      VENT_PACE_CTRL = 1;
    (default) -> VOO_Charging
    VOO_Charging -> VOO_Pacing : after(lowrateInterval - vPaceWidth, msec)
    VOO_Pacing -> VOO_Charging : after(vPaceWidth, msec)
  state AAI
    state pARP
      %atrial refractory period from paced beat
      entry:
      FRONTEND_CTRL = 1;
      PACING_REF_PWM = aPaceAmp;
      PACE_GND_CTRL=1;
      ATR_PACE_CTRL = 0;
      PACE_CHARGE_CTRL = 1;
      ATR_GND_CTRL = 1;
    state pReady
      %refratory period
      %finishes after
      %paced beat
    state Discharging
      %discharging
      entry:
      PACE_CHARGE_CTRL = 0;
      ATR_GND_CTRL = 0;
      ATR_PACE_CTRL = 1;
    state sARP
      %atrial refractory
      %period from
      %sensed beat
    state sReady
      %refratory period
      %finishes after
      %sensed beat
    AAI.Discharging -> AAI.pARP : after(aPaceWidth, msec)
    (default) -> AAI.pARP
    AAI.pARP -> AAI.pReady : after(ARP - aPaceWidth,  msec)
    AAI.pReady -> AAI.Discharging [order 1] : after(lowrateInterval - ARP, msec)
    AAI.pReady -> AAI.sARP [order 2] : [ATR_CMP_DETECT]
    AAI.sReady -> AAI.Discharging [order 1] : after(lowrateInterval - ARP + (hysteresis * hysteresisInterval), msec)
    AAI.sARP -> AAI.sReady : after(ARP, msec)
    AAI.sReady -> AAI.sARP [order 2] : [ATR_CMP_DETECT]
  state VVI
    state pVRP
      %ventricular refractory period from paced beat
      entry:
      FRONTEND_CTRL = 1;
      PACING_REF_PWM = vPaceAmp;
      PACE_GND_CTRL=1;
      VENT_PACE_CTRL = 0;
      PACE_CHARGE_CTRL = 1;
      VENT_GND_CTRL = 1;
    state Discharging
      %discharging
      entry:
      PACE_CHARGE_CTRL = 0;
      VENT_GND_CTRL = 0;
      VENT_PACE_CTRL = 1;
    state pReady
      %refratory period
      %finishes after
      %paced beat
    state sVRP
      %atrial refractory
      %period from
      %sensed beat
    state sReady
      %refratory period
      %finishes after
      %sensed beat
    VVI.Discharging -> VVI.pVRP : after(vPaceWidth, msec)
    (default) -> VVI.pVRP
    VVI.pVRP -> VVI.pReady : after(VRP - vPaceWidth, msec)
    VVI.pReady -> VVI.Discharging [order 1] : after(lowrateInterval - VRP, msec)
    VVI.pReady -> VVI.sVRP [order 2] : [VENT_CMP_DETECT]
    VVI.sReady -> VVI.Discharging [order 1] : after(lowrateInterval - VRP + (hysteresis * hysteresisInterval), msec)
    VVI.sVRP -> VVI.sReady : after(VRP, msec)
    VVI.sReady -> VVI.sVRP [order 2] : [VENT_CMP_DETECT]
  state AOOR
    state AOOR_Charging
      %charging capacitor
      entry:
      PACING_REF_PWM = aPaceAmp;
      PACE_GND_CTRL = 1;
      Z_ATR_CTRL = 0;
      ATR_PACE_CTRL = 0;
      PACE_CHARGE_CTRL = 1;
      ATR_GND_CTRL = 1;
    state AOOR_Pacing
      %discharging
      entry:
      Z_ATR_CTRL = 1;
      PACE_CHARGE_CTRL = 0;
      ATR_GND_CTRL = 0;
      ATR_PACE_CTRL = 1;
    (default) -> AOOR_Charging
    AOOR_Charging -> AOOR_Pacing : after(rate_adapt_interval - aPaceWidth, msec)
    AOOR_Pacing -> AOOR_Charging : after(aPaceWidth, msec)
  state VOOR
    state VOOR_Charging
      %charging capacitor
      entry:
      PACING_REF_PWM = vPaceAmp;
      PACE_GND_CTRL = 1;
      Z_VENT_CTRL = 0;
      VENT_PACE_CTRL = 0;
      PACE_CHARGE_CTRL = 1;
      VENT_GND_CTRL = 1;
    state VOOR_Pacing
      %discharging capacitor
      entry:
      Z_VENT_CTRL = 1;
      PACE_CHARGE_CTRL = 0;
      VENT_GND_CTRL = 0;
      VENT_PACE_CTRL = 1;
    (default) -> VOOR_Charging
    VOOR_Charging -> VOOR_Pacing : after(rate_adapt_interval - vPaceWidth, msec)
    VOOR_Pacing -> VOOR_Charging : after(vPaceWidth,msec)
  state AAIR
    state pARP
      %atrial refractory period from paced beat
      entry:
      FRONTEND_CTRL = 1;
      PACING_REF_PWM = aPaceAmp;
      PACE_GND_CTRL=1;
      ATR_PACE_CTRL = 0;
      PACE_CHARGE_CTRL = 1;
      ATR_GND_CTRL = 1;
    state pReady
      %refratory period
      %finishes after
      %paced beat
    state Discharging
      %discharging
      entry:
      PACE_CHARGE_CTRL = 0;
      ATR_GND_CTRL = 0;
      ATR_PACE_CTRL = 1;
    state sARP
      %atrial refractory
      %period from
      %sensed beat
    state sReady
      %refratory period
      %finishes after
      %sensed beat
    AAIR.Discharging -> AAIR.pARP : after(aPaceWidth, msec)
    (default) -> AAIR.pARP
    AAIR.pARP -> AAIR.pReady : after(ARP- aPaceWidth,  msec)
    AAIR.pReady -> AAIR.Discharging [order 1] : after(rate_adapt_interval - ARP , msec)
    AAIR.pReady -> AAIR.sARP [order 2] : [ATR_CMP_DETECT]
    AAIR.sReady -> AAIR.Discharging [order 1] : after(rate_adapt_interval - ARP + (hysteresis * hysteresisInterval), msec)
    AAIR.sARP -> AAIR.sReady : after(ARP, msec)
    AAIR.sReady -> AAIR.sARP [order 2] : [ATR_CMP_DETECT]
  state VVIR
    state pVRP
      %ventricular refractory period from paced beat
      entry:
      FRONTEND_CTRL = 1;
      PACING_REF_PWM = vPaceAmp;
      PACE_GND_CTRL=1;
      VENT_PACE_CTRL = 0;
      PACE_CHARGE_CTRL = 1;
      VENT_GND_CTRL = 1;
    state Discharging
      %discharging
      entry:
      PACE_CHARGE_CTRL = 0;
      VENT_GND_CTRL = 0;
      VENT_PACE_CTRL = 1;
    state pReady
      %refratory period
      %finishes after
      %paced beat
    state sVRP
      %atrial refractory
      %period from
      %sensed beat
    state sReady
      %refratory period
      %finishes after
      %sensed beat
    VVIR.Discharging -> VVIR.pVRP : after(vPaceWidth, msec)
    (default) -> VVIR.pVRP
    VVIR.pVRP -> VVIR.pReady : after(VRP - vPaceWidth, msec)
    VVIR.pReady -> VVIR.Discharging [order 1] : after(rate_adapt_interval - VRP, msec)
    VVIR.pReady -> VVIR.sVRP [order 2] : [VENT_CMP_DETECT]
    VVIR.sReady -> VVIR.Discharging [order 1] : after(rate_adapt_interval - VRP + (hysteresis * hysteresisInterval), msec)
    VVIR.sVRP -> VVIR.sReady : after(VRP, msec)
    VVIR.sReady -> VVIR.sVRP [order 2] : [VENT_CMP_DETECT]
  INIT -> AOO [order 1] : [mode == 0]
  AOO -> INIT : [mode ~=0]
  INIT -> VOO [order 2] : [mode==1]
  VOO -> INIT : [mode~=1]
  INIT -> AAI [order 3] : [mode == 2]
  AAI -> INIT : [mode ~=2]
  INIT -> VVI [order 4] : [mode==3]
  VVI -> INIT : [mode~=3]
  INIT -> AOOR [order 5] : [mode==4]
  AOOR -> INIT : [mode~=4]
  (default) -> INIT
  INIT -> VOOR [order 6] : [mode==5]
  VOOR -> INIT : [mode~=5]
  INIT -> AAIR [order 7] : [mode==6]
  AAIR -> INIT : [mode~=6]
  INIT -> VVIR [order 8] : [mode==7]
  VVIR -> INIT : [mode~=7]
  data: VENT_CMP_DETECT input; ATR_CMP_DETECT input; ATR_GND_CTRL output; ATR_PACE_CTRL output; PACE_CHARGE_CTRL output; VENT_GND_CTRL output; VENT_PACE_CTRL output; Z_ATR_CTRL output; aPaceAmp input; vPaceAmp input; aPaceWidth input; vPaceWidth input; ARP input; VRP input; lowrateInterval input; a_sense input; v_sense input; mode input; Z_VENT_CTRL output; PACING_REF_PWM output; PACE_GND_CTRL output; FRONTEND_CTRL output; VENT_CMP_REF_PWM output; ATR_CMP_REF_PWM output; hysteresisInterval input; hysteresis input; rate_adapt_interval input

== stateflow chart Deliverable2_SimulinkModel_Group37_Demo/Subsystem1/Chart ==
  state ACTIVE
    entry:
    controlled_vent = VENT_PACE_CTRL
  state BLOCKED
    entry:
    controlled_vent = 0
  (default) -> ACTIVE
  BLOCKED -> BLOCKED [order 2]
  ACTIVE -> ACTIVE [order 2]
  ACTIVE -> BLOCKED [order 1] : [butt_push ==1]
  BLOCKED -> ACTIVE [order 1] : [butt_push~=1]
  data: butt_push input; VENT_PACE_CTRL input; controlled_vent output

== stateflow chart Deliverable2_SimulinkModel_Group37_Demo/Subsystem3/Chart ==
  state PARAMETER_SETTING
    mode=rxdata(3);
    A_pulse_width=rxdata(4);
    V_pulse_width=rxdata(5);
    lower_rate_limit=rxdata(6);
    A_amp=rxdata(7);
    V_amp=rxdata(8);
    A_refractory=rxdata(9);
    V_refractory=rxdata(10);
    A_sensitivity=rxdata(11);
    V_sensitivity=rxdata(12);
    recovery_time=rxdata(13);
    response_factor=rxdata(14);
    max_sensor_rate=rxdata(15);
    activity_threshold=rxdata(16);
    reaction_time=rxdata(17);
    hysterisis=rxdata(18);
  state INITAL
    entry:
    mode=0;
    lower_rate_limit = 60;
    A_pulse_width=100;
    V_pulse_width=100;
    A_amp=35;
    V_amp=35;
    A_refractory=25;
    V_refractory=32;
    activity_threshold=20;
    reaction_time=30;
    A_sensitivity=35;
    V_sensitivity=35;
    recovery_time=5;
    response_factor=8;
    max_sensor_rate=120;
    hysterisis = 0;
  state STANDBY
  state SENDING_PARAMS
    entry:
    send_params();
  PARAMETER_SETTING -> STANDBY
  (default) -> INITAL
  (junction 7) -> PARAMETER_SETTING [order 1] : [rxdata(2)==hex2dec('55')]
  (junction 34) -> STANDBY [order 2] : [status == 0]
  INITAL -> STANDBY
  STANDBY -> (junction 34)
  (junction 34) -> (junction 7) [order 1] : [rxdata(1)==hex2dec('16')]
  (junction 7) -> SENDING_PARAMS [order 2] : [rxdata(2)==hex2dec('22')]
  SENDING_PARAMS -> STANDBY
  data: rxdata input; status input; mode output; response_factor output; recovery_time output; reaction_time output; max_sensor_rate output; lower_rate_limit output; activity_threshold output; V_sensitivity output; V_refractory output; V_pulse_width output; V_amp output; A_sensitivity output; A_refractory output; A_pulse_width output; A_amp output; hysterisis output

== stateflow chart Deliverable2_SimulinkModel_Group37_Demo/Subsystem6/Subsystem5/Chart1 ==
  settings: sampleTime=0.001
  state Reset
  state Rate_Adapt
    state ACCELERATION
      entry:
      new_pacing_rate = current_pacing_rate + (maximum_sensor_rate - lowRate) / (reaction_time*1000)
      if new_pacing_rate >= maximum_sensor_rate
      new_pacing_rate = maximum_sensor_rate
      end
    state INIT
      entry:
      new_pacing_rate = lowRate;
    state STEADY
      entry:
      new_pacing_rate = current_pacing_rate;
    state DEACCELERATION
      entry:
      new_pacing_rate = current_pacing_rate - (maximum_sensor_rate - lowRate) / (recovery_time*1000)
      if new_pacing_rate <= lowRate
      new_pacing_rate = lowRate
      end
    ACCELERATION -> ACCELERATION [order 3] : after(1,msec)
    (default) -> INIT
    STEADY -> ACCELERATION [order 1] : [desired_pacing_rate>current_pacing_rate]
    ACCELERATION -> STEADY [order 1] : [desired_pacing_rate==current_pacing_rate]
    DEACCELERATION -> ACCELERATION [order 2] : [desired_pacing_rate>current_pacing_rate]
    ACCELERATION -> DEACCELERATION [order 2] : [desired_pacing_rate<current_pacing_rate]
    INIT -> STEADY
    STEADY -> DEACCELERATION [order 2] : [desired_pacing_rate<current_pacing_rate]
    DEACCELERATION -> STEADY [order 1] : [desired_pacing_rate==current_pacing_rate]
    DEACCELERATION -> DEACCELERATION [order 3] : after(1,msec)
  (default) -> Reset
  Reset -> Rate_Adapt
  Rate_Adapt -> Reset : [mode~=last_mode]
  data: mode input; last_mode input; current_pacing_rate input; reaction_time input; recovery_time input; desired_pacing_rate input; lowRate input; maximum_sensor_rate input; new_pacing_rate output double
